simulink model "Active_mass_suspension"  (R2023a)
settings: Solver=VariableStepAuto  StartTime=0.0  StopTime=10  RelTol=1e-3
libraries: fuzblock x2, slpidlib x2, mpclib x1
settings Model: Creator=SAGNEEK SENGUPTA  LastModifiedBy=SAGNEEK SENGUPTA

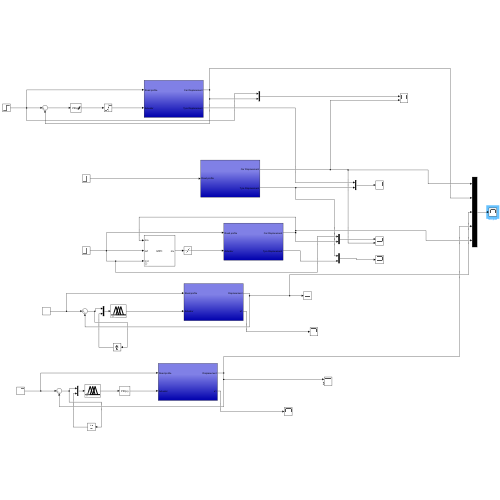
[thumbnail: Simulink's stored preview of the top-level diagram]
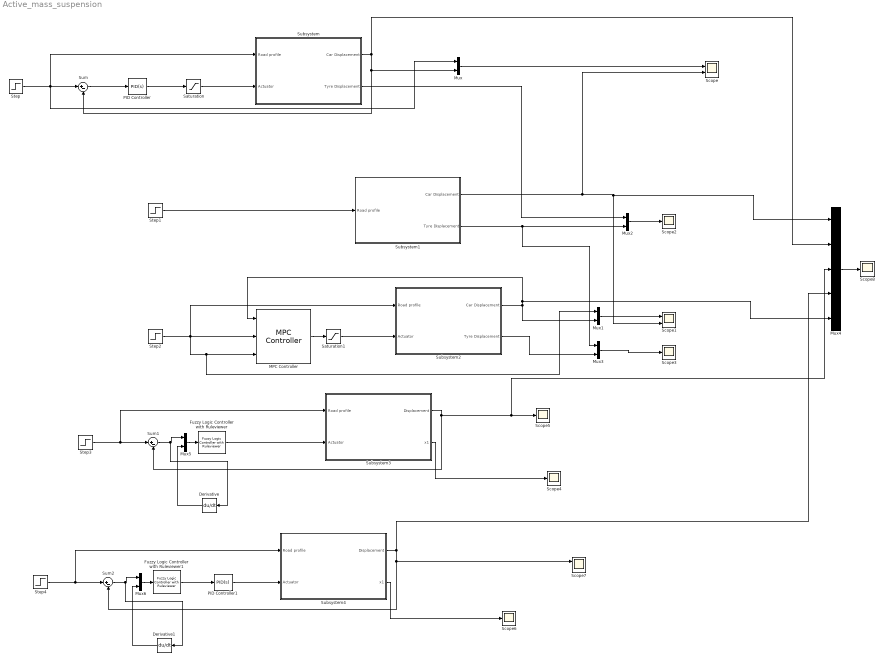
== system Active_mass_suspension ==
  Derivative : Derivative
  Derivative1 : Derivative
  Fuzzy Logic Controller with Ruleviewer : fuzblock/Fuzzy Logic  Controller  with Ruleviewer  fismatrix=rules_3  Ts=2
  Fuzzy Logic Controller with Ruleviewer1 : fuzblock/Fuzzy Logic  Controller  with Ruleviewer  fismatrix=rules_3  Ts=2
  MPC Controller : mpclib/MPC Controller  SCDEnableBlockLinearizationSpecification=on  mpcobj=mpc1  is_multiple=0  enable_value=0  return_u0=off  updateMPCinCallerWorkspace=on  md_inport=on  mv_inport=off  uref_inport=off  return_cost=off  return_mvseq=off  return_qpstatus=off  return_xseq=off  return_state=off  return_ovseq=off  state_inport=off  umin_inport=off  umax_inport=off  ymin_inport=off  ymax_inport=off  cc_inport=off  ywt_inport=off  uwt_inport=off  duwt_inport=off  rhoeps_inport=off  pm_inport=off  MaximumP=10  HorizonChoice=FixedHorizon  n_ts=0.01  n_p=12  n_mv=1  n_md=1  n_ud=0  n_mo=1  n_uo=0  BlockDataType=double  SampleTimeInherited=off  switch_inport=off
  Mux{,1..3,5..6} (6 alike) : Mux  Inputs=2
  Mux4 : Mux  Inputs=5
  PID Controller : slpidlib/PID Controller  Controller=PID  Form=Parallel  TimeDomain=Continuous-time  UseExternalTs=off  SampleTime=-1  IntegratorMethod=Forward Euler  FilterMethod=Forward Euler  ControllerParametersSource=internal  P=100  I=900  UseKiTs=on  D=80  N=1000  UseFilter=on  TunerSelectOption=Frequency Response Based  InitialConditionSource=internal  InitialConditionForIntegrator=0  InitialConditionForFilter=0  DifferentiatorICPrevScaledInput=0  ExternalReset=none  TrackingMode=off  Kt=1  LimitOutput=on  SatLimitsSource=internal  UpperSaturationLimit=800  LowerSaturationLimit=-800  LinearizeAsGain=on  AntiWindupMode=none  Kb=1  LimitIntegrator=off  UpperIntegratorSaturationLimit=inf  LowerIntegratorSaturationLimit=-inf  POutMin=[]  POutMax=[]  IOutMin=[]  IOutMax=[]  DOutMin=[]  DOutMax=[]  NOutMin=[]  NOutMax=[]  SumOutMin=[]  SumOutMax=[]  SaturationOutMin=[]  SaturationOutMax=[]  PParamMin=[]  PParamMax=[]  IParamMin=[]  IParamMax=[]  DParamMin=[]  DParamMax=[]  NParamMin=[]  NParamMax=[]  KbParamMin=[]  KbParamMax=[]  KtParamMin=[]  KtParamMax=[]  KbOutMin=[]  KbOutMax=[]  KtOutMin=[]  KtOutMax=[]  IntegratorOutMin=[]  IntegratorOutMax=[]  FilterOutMin=[]  FilterOutMax=[]  SumI1OutMin=[]  SumI1OutMax=[]  SumI2OutMin=[]  SumI2OutMax=[]  SumI3OutMin=[]  SumI3OutMax=[]  SumI4OutMin=[]  SumI4OutMax=[]  SumDOutMin=[]  SumDOutMax=[]  DifferentiatorOutMin=[]  DifferentiatorOutMax=[]  FilterDiffOutCoefMin=[]  FilterDiffOutCoefMax=[]  ReciprocalOutMin=[]  ReciprocalOutMax=[]  SumDenOutMin=[]  SumDenOutMax=[]  SumNumOutMin=[]  SumNumOutMax=[]  DivideOutMin=[]  DivideOutMax=[]  UdiffTsProdOutMin=[]  UdiffTsProdOutMax=[]  NTsProdOutMin=[]  NTsProdOutMax=[]  UintegralTsProdOutMin=[]  UintegralTsProdOutMax=[]  UngainTsProdOutMin=[]  UngainTsProdOutMax=[]  ClampingZeroOutDataTypeStr=Inherit: Inherit via back propagation  ClampingZeroOutMin=[]  ClampingZeroOutMax=[]  FilterDenConstantOutDataTypeStr=Inherit: Inherit via back propagation  FilterDenConstantOutMin=[]  FilterDenConstantOutMax=[]  PCopyOutDataTypeStr=Inherit: Inherit via back propagation  PCopyOutMin=[]  PCopyOutMax=[]  NCopyOutDataTypeStr=Inherit: Inherit via back propagation  NCopyOutMin=[]  NCopyOutMax=[]  IntegratorContinuousStateAttributes=''  IntegratorStateMustResolveToSignalObject=off  IntegratorRTWStateStorageClass=Auto  FilterContinuousStateAttributes=''  FilterStateMustResolveToSignalObject=off  FilterRTWStateStorageClass=Auto  ParallelPVariant=InternalParameters  IdealPVariant=Disabled  IVariant=InternalParameters  DVariant=InternalParameters  IntegratorVariant=Continuous  SatVariant=Enabled  AWVariant=Passthrough  PCopyVariant=Disabled  TRVariant=Disabled  FdbkBlocksVariant=Forward  IdealPFdbkVariant=Disabled  SatFdbkVariant=Disabled  DerivativeFilterVariant=ContFilter  NVariant=InternalParameters  NCopyVariant=Disabled  FilterICVariant=InternalICsFilter  IntegratorICVariant=InternalICs  ExternalResetVariant=Disabled  TRSumVariant=Passthrough  SumFdbkVariant=Disabled  SumVariant=Sum_PID  TsampFilterVariant=InternalTs  TsampNgainVariant=Passthrough  TsampIntegralVariant=Disabled_SignalSpec  ExternalSaturationOutDataTypeStr=Inherit: Same as second input
  PID Controller1 : slpidlib/PID Controller  Controller=PID  Form=Parallel  TimeDomain=Continuous-time  UseExternalTs=off  SampleTime=-1  IntegratorMethod=Forward Euler  FilterMethod=Forward Euler  ControllerParametersSource=internal  P=20  I=600  UseKiTs=off  D=0.1  N=100  UseFilter=on  TunerSelectOption=Transfer Function Based (PID Tuner App)  InitialConditionSource=internal  InitialConditionForIntegrator=0  InitialConditionForFilter=0  DifferentiatorICPrevScaledInput=0  ExternalReset=none  TrackingMode=off  Kt=1  LimitOutput=off  SatLimitsSource=internal  UpperSaturationLimit=inf  LowerSaturationLimit=-inf  LinearizeAsGain=on  AntiWindupMode=none  Kb=1  LimitIntegrator=off  UpperIntegratorSaturationLimit=inf  LowerIntegratorSaturationLimit=-inf  POutMin=[]  POutMax=[]  IOutMin=[]  IOutMax=[]  DOutMin=[]  DOutMax=[]  NOutMin=[]  NOutMax=[]  SumOutMin=[]  SumOutMax=[]  SaturationOutMin=[]  SaturationOutMax=[]  PParamMin=[]  PParamMax=[]  IParamMin=[]  IParamMax=[]  DParamMin=[]  DParamMax=[]  NParamMin=[]  NParamMax=[]  KbParamMin=[]  KbParamMax=[]  KtParamMin=[]  KtParamMax=[]  KbOutMin=[]  KbOutMax=[]  KtOutMin=[]  KtOutMax=[]  IntegratorOutMin=[]  IntegratorOutMax=[]  FilterOutMin=[]  FilterOutMax=[]  SumI1OutMin=[]  SumI1OutMax=[]  SumI2OutMin=[]  SumI2OutMax=[]  SumI3OutMin=[]  SumI3OutMax=[]  SumI4OutMin=[]  SumI4OutMax=[]  SumDOutMin=[]  SumDOutMax=[]  DifferentiatorOutMin=[]  DifferentiatorOutMax=[]  FilterDiffOutCoefMin=[]  FilterDiffOutCoefMax=[]  ReciprocalOutMin=[]  ReciprocalOutMax=[]  SumDenOutMin=[]  SumDenOutMax=[]  SumNumOutMin=[]  SumNumOutMax=[]  DivideOutMin=[]  DivideOutMax=[]  UdiffTsProdOutMin=[]  UdiffTsProdOutMax=[]  NTsProdOutMin=[]  NTsProdOutMax=[]  UintegralTsProdOutMin=[]  UintegralTsProdOutMax=[]  UngainTsProdOutMin=[]  UngainTsProdOutMax=[]  ClampingZeroOutDataTypeStr=Inherit: Inherit via back propagation  ClampingZeroOutMin=[]  ClampingZeroOutMax=[]  FilterDenConstantOutDataTypeStr=Inherit: Inherit via back propagation  FilterDenConstantOutMin=[]  FilterDenConstantOutMax=[]  PCopyOutDataTypeStr=Inherit: Inherit via back propagation  PCopyOutMin=[]  PCopyOutMax=[]  NCopyOutDataTypeStr=Inherit: Inherit via back propagation  NCopyOutMin=[]  NCopyOutMax=[]  IntegratorContinuousStateAttributes=''  IntegratorStateMustResolveToSignalObject=off  IntegratorRTWStateStorageClass=Auto  FilterContinuousStateAttributes=''  FilterStateMustResolveToSignalObject=off  FilterRTWStateStorageClass=Auto  ParallelPVariant=InternalParameters  IdealPVariant=Disabled  IVariant=InternalParameters  DVariant=InternalParameters  IntegratorVariant=Continuous  SatVariant=Disabled  AWVariant=Passthrough  PCopyVariant=Disabled  TRVariant=Disabled  FdbkBlocksVariant=Forward  IdealPFdbkVariant=Disabled  SatFdbkVariant=Disabled  DerivativeFilterVariant=ContFilter  NVariant=InternalParameters  NCopyVariant=Disabled  FilterICVariant=InternalICsFilter  IntegratorICVariant=InternalICs  ExternalResetVariant=Disabled  TRSumVariant=Passthrough  SumFdbkVariant=Disabled  SumVariant=Sum_PID  TsampFilterVariant=InternalTs  TsampNgainVariant=Passthrough  TsampIntegralVariant=Disabled_SignalSpec  ExternalSaturationOutDataTypeStr=Inherit: Same as second input
  Saturation : Saturate  UpperLimit=800  LowerLimit=-800
  Saturation1 : Saturate  UpperLimit=800  LowerLimit=-800
  Scope : Scope  NumInputPorts=2
  Scope1 : Scope  NumInputPorts=2
  Scope{2..6,8} (6 alike) : Scope
  Scope7 : Scope  NumInputPorts=2
  Step{,1..4} (5 alike) : Step  Time=0  SampleTime=0
  Subsystem : Subsystem
  Subsystem1 : Subsystem
  Subsystem2 : Subsystem
  Subsystem3 : Subsystem
  Subsystem4 : Subsystem
  Sum : Sum  Inputs=|+-
  Sum1 : Sum  Inputs=|+-
  Sum2 : Sum  Inputs=|+-
  wires:
  Step/1 -> Subsystem/1(Road profile), Sum/1, Mux/1
  Saturation/1 -> Subsystem/2(Actuator)
  Subsystem/1(Car Displacement) -> Sum/2, Mux/2, Mux4/2
  Mux/1 -> Scope/1
  Step1/1 -> Subsystem1/1(Road profile)
  Subsystem1/1(Car Displacement) -> Mux4/1, Scope1/2, Scope/2
  PID Controller/1 -> Saturation/1
  Sum/1 -> PID Controller/1
  Saturation1/1 -> Subsystem2/2(Actuator)
  Subsystem2/1(Car Displacement) -> Mux1/2, Mux4/5, MPC Controller/1
  Mux1/1 -> Scope1/1
  MPC Controller/1 -> Saturation1/1
  Step2/1 -> MPC Controller/2, Mux1/1, MPC Controller/3, Subsystem2/1(Road profile)
  Subsystem1/2(Tyre Displacement) -> Mux3/1, Mux2/2
  Subsystem/2(Tyre Displacement) -> Mux2/1
  Mux2/1 -> Scope2/1
  Subsystem2/2(Tyre Displacement) -> Mux3/2
  Mux3/1 -> Scope3/1
  Subsystem4/1(Displacement) -> Scope7/1, Sum2/2, Mux4/4
  Derivative1/1 -> Mux6/2
  Step4/1 -> Subsystem4/1(Road profile), Sum2/1
  Mux6/1 -> Fuzzy Logic Controller with Ruleviewer1/1
  Fuzzy Logic Controller with Ruleviewer1/1 -> PID Controller1/1
  PID Controller1/1 -> Subsystem4/2(Actuator)
  Sum2/1 -> Derivative1/1, Mux6/1
  Subsystem4/2(x1) -> Scope6/1
  Fuzzy Logic Controller with Ruleviewer/1 -> Subsystem3/2(Actuator)
  Subsystem3/2(x1) -> Scope4/1
  Step3/1 -> Subsystem3/1(Road profile), Sum1/1
  Subsystem3/1(Displacement) -> Mux4/3, Scope5/1, Sum1/2
  Derivative/1 -> Mux5/2
  Sum1/1 -> Derivative/1, Mux5/1
  Mux5/1 -> Fuzzy Logic Controller with Ruleviewer/1
  Mux4/1 -> Scope8/1

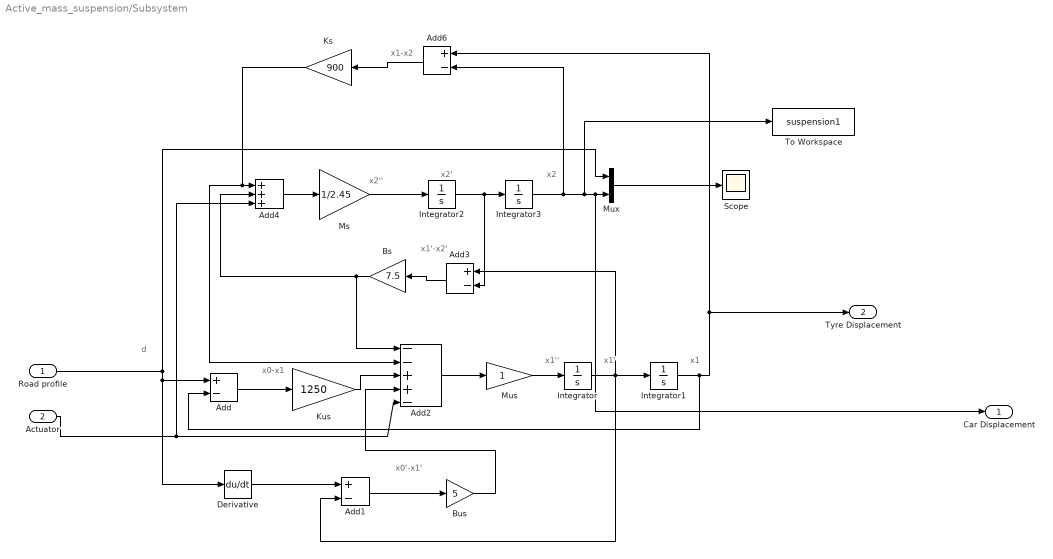
== system Active_mass_suspension/Subsystem ==
  note: x0-x1
  note: x0'-x1'
  note: x1
  note: x1'
  note: x2'
  note: x2''
  note: d
  note: x1'-x2'
  note: x1-x2
  note: x2
  note: x1''
  Road profile : Inport
  Actuator : Inport  Port=2
  Add{,1,3,6} (4 alike) : Sum  Inputs=+-
  Add2 : Sum  Inputs=--++-
  Add4 : Sum  Inputs=+++
  Bs : Gain  Gain=7.5
  Bus : Gain  Gain=5
  Derivative : Derivative
  Integrator{,1..3} (4 alike) : Integrator
  Ks : Gain  Gain=900
  Kus : Gain  Gain=1250
  Ms : Gain  Gain=1/2.45
  Mus : Gain
  Mux : Mux  Inputs=2
  Scope : Scope
  To Workspace : ToWorkspace  VariableName=suspension1  SaveFormat=Timeseries  SampleTime=-1
  Car Displacement : Outport
  Tyre Displacement : Outport  Port=2
  wires:
  Integrator1/1 -> Add/2, Tyre Displacement/1, Add6/1
  Bs/1 -> Add4/2, Add2/1
  Ms/1 -> Integrator2/1
  Bus/1 -> Add2/4
  Actuator/1 -> Add4/3, Add2/5
  Kus/1 -> Add2/3
  Integrator3/1 -> Car Displacement/1, Mux/2, To Workspace/1, Add6/2
  Add/1 -> Kus/1
  Mus/1 -> Integrator/1
  Ks/1 -> Add2/2, Add4/1
  Mux/1 -> Scope/1
  Add3/1 -> Bs/1
  Integrator2/1 -> Add3/2, Integrator3/1
  Add1/1 -> Bus/1
  Derivative/1 -> Add1/1
  Add2/1 -> Mus/1
  Integrator/1 -> Add1/2, Add3/1, Integrator1/1
  Add4/1 -> Ms/1
  Road profile/1 -> Derivative/1, Add/1, Mux/1
  Add6/1 -> Ks/1

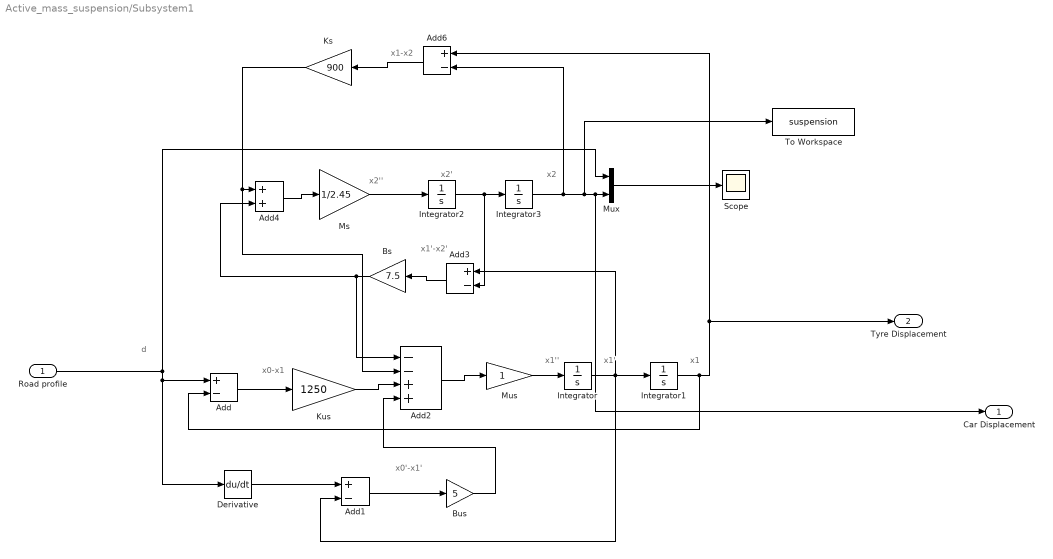
== system Active_mass_suspension/Subsystem1 ==
  note: x0-x1
  note: x0'-x1'
  note: x1
  note: x1'
  note: x2'
  note: x2''
  note: d
  note: x1'-x2'
  note: x1-x2
  note: x2
  note: x1''
  Road profile : Inport
  Add{,1,3,6} (4 alike) : Sum  Inputs=+-
  Add2 : Sum  Inputs=--++
  Add4 : Sum
  Bs : Gain  Gain=7.5
  Bus : Gain  Gain=5
  Derivative : Derivative
  Integrator{,1..3} (4 alike) : Integrator
  Ks : Gain  Gain=900
  Kus : Gain  Gain=1250
  Ms : Gain  Gain=1/2.45
  Mus : Gain
  Mux : Mux  Inputs=2
  Scope : Scope
  To Workspace : ToWorkspace  VariableName=suspension  SaveFormat=Timeseries  SampleTime=-1
  Car Displacement : Outport
  Tyre Displacement : Outport  Port=2
  wires:
  Integrator1/1 -> Add/2, Tyre Displacement/1, Add6/1
  Bs/1 -> Add4/2, Add2/1
  Ms/1 -> Integrator2/1
  Bus/1 -> Add2/4
  Kus/1 -> Add2/3
  Integrator3/1 -> Car Displacement/1, Mux/2, To Workspace/1, Add6/2
  Add/1 -> Kus/1
  Mus/1 -> Integrator/1
  Ks/1 -> Add2/2, Add4/1
  Mux/1 -> Scope/1
  Add3/1 -> Bs/1
  Integrator2/1 -> Add3/2, Integrator3/1
  Add1/1 -> Bus/1
  Derivative/1 -> Add1/1
  Add2/1 -> Mus/1
  Integrator/1 -> Add1/2, Add3/1, Integrator1/1
  Add4/1 -> Ms/1
  Road profile/1 -> Derivative/1, Add/1, Mux/1
  Add6/1 -> Ks/1

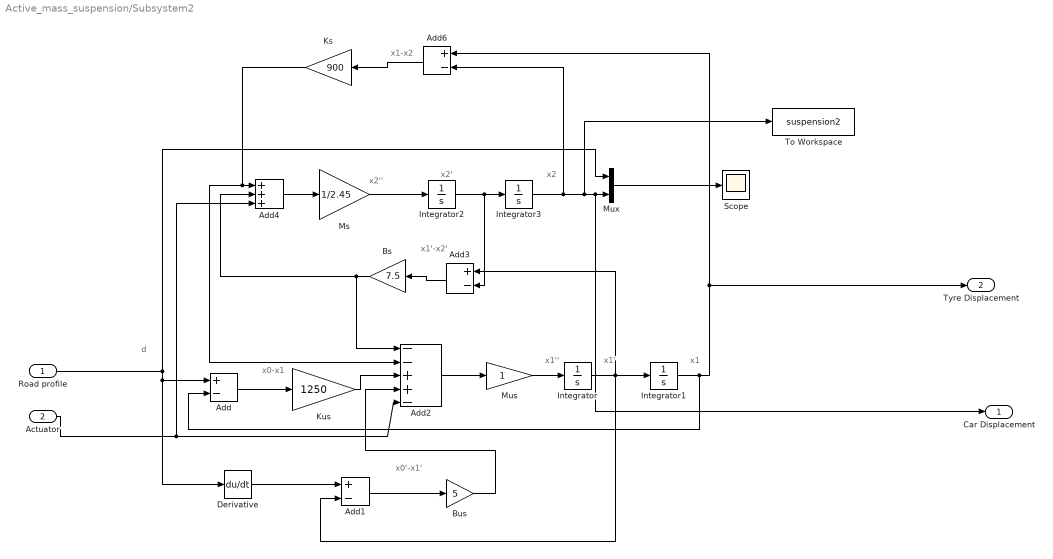
== system Active_mass_suspension/Subsystem2 ==
  note: x0-x1
  note: x0'-x1'
  note: x1
  note: x1'
  note: x2'
  note: x2''
  note: d
  note: x1'-x2'
  note: x1-x2
  note: x2
  note: x1''
  Road profile : Inport
  Actuator : Inport  Port=2
  Add{,1,3,6} (4 alike) : Sum  Inputs=+-
  Add2 : Sum  Inputs=--++-
  Add4 : Sum  Inputs=+++
  Bs : Gain  Gain=7.5
  Bus : Gain  Gain=5
  Derivative : Derivative
  Integrator{,1..3} (4 alike) : Integrator
  Ks : Gain  Gain=900
  Kus : Gain  Gain=1250
  Ms : Gain  Gain=1/2.45
  Mus : Gain
  Mux : Mux  Inputs=2
  Scope : Scope
  To Workspace : ToWorkspace  VariableName=suspension2  SaveFormat=Timeseries  SampleTime=-1
  Car Displacement : Outport
  Tyre Displacement : Outport  Port=2
  wires:
  Integrator1/1 -> Add/2, Tyre Displacement/1, Add6/1
  Bs/1 -> Add4/2, Add2/1
  Ms/1 -> Integrator2/1
  Bus/1 -> Add2/4
  Actuator/1 -> Add4/3, Add2/5
  Kus/1 -> Add2/3
  Integrator3/1 -> Car Displacement/1, Mux/2, To Workspace/1, Add6/2
  Add/1 -> Kus/1
  Mus/1 -> Integrator/1
  Ks/1 -> Add2/2, Add4/1
  Mux/1 -> Scope/1
  Add3/1 -> Bs/1
  Integrator2/1 -> Add3/2, Integrator3/1
  Add1/1 -> Bus/1
  Derivative/1 -> Add1/1
  Add2/1 -> Mus/1
  Integrator/1 -> Add1/2, Add3/1, Integrator1/1
  Add4/1 -> Ms/1
  Road profile/1 -> Derivative/1, Add/1, Mux/1
  Add6/1 -> Ks/1

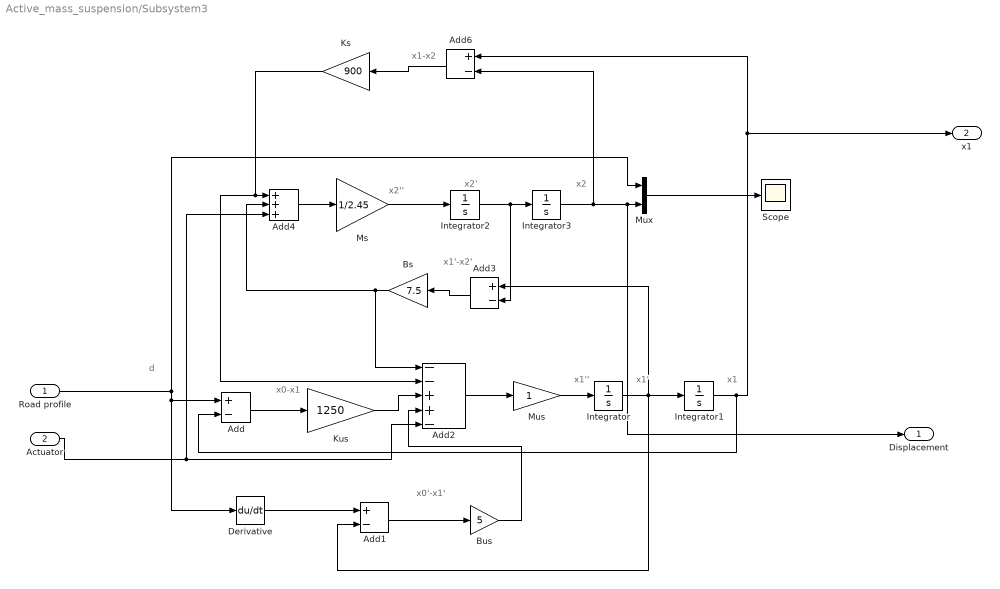
== system Active_mass_suspension/Subsystem3 ==
  note: x0-x1
  note: x0'-x1'
  note: x1
  note: x1'
  note: x2'
  note: x2''
  note: d
  note: x1'-x2'
  note: x1-x2
  note: x2
  note: x1''
  Road profile : Inport
  Actuator : Inport  Port=2
  Add{,1,3,6} (4 alike) : Sum  Inputs=+-
  Add2 : Sum  Inputs=--++-
  Add4 : Sum  Inputs=+++
  Bs : Gain  Gain=7.5
  Bus : Gain  Gain=5
  Derivative : Derivative
  Integrator{,1..3} (4 alike) : Integrator
  Ks : Gain  Gain=900
  Kus : Gain  Gain=1250
  Ms : Gain  Gain=1/2.45
  Mus : Gain
  Mux : Mux  Inputs=2
  Scope : Scope
  Displacement : Outport
  x1 : Outport  Port=2
  wires:
  Integrator1/1 -> Add/2, x1/1, Add6/1
  Bs/1 -> Add4/2, Add2/1
  Ms/1 -> Integrator2/1
  Bus/1 -> Add2/4
  Actuator/1 -> Add4/3, Add2/5
  Kus/1 -> Add2/3
  Integrator3/1 -> Displacement/1, Mux/2, Add6/2
  Add/1 -> Kus/1
  Mus/1 -> Integrator/1
  Ks/1 -> Add2/2, Add4/1
  Mux/1 -> Scope/1
  Add3/1 -> Bs/1
  Integrator2/1 -> Add3/2, Integrator3/1
  Add1/1 -> Bus/1
  Derivative/1 -> Add1/1
  Add2/1 -> Mus/1
  Integrator/1 -> Add1/2, Add3/1, Integrator1/1
  Add4/1 -> Ms/1
  Road profile/1 -> Derivative/1, Add/1, Mux/1
  Add6/1 -> Ks/1

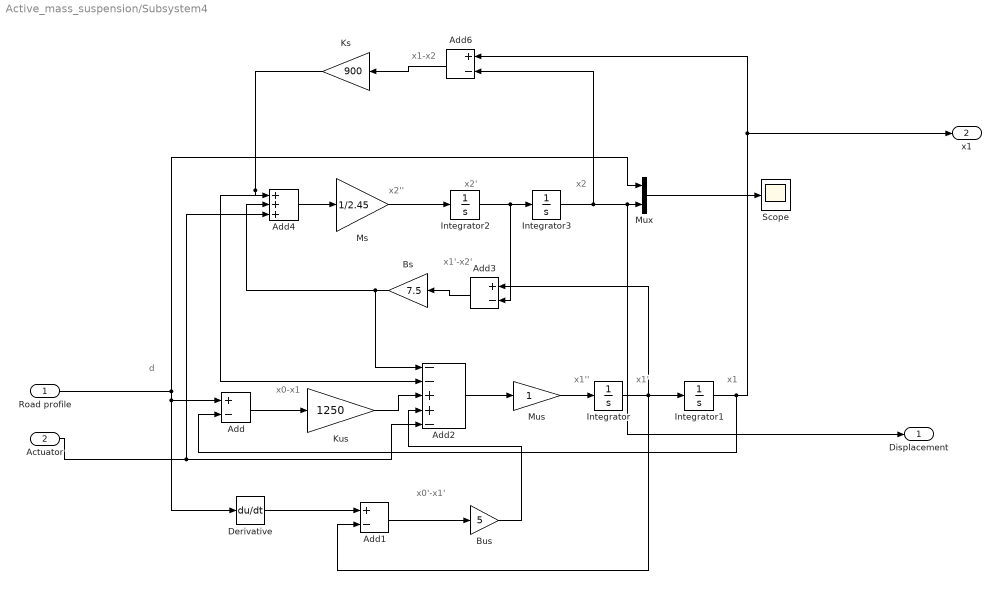
== system Active_mass_suspension/Subsystem4 ==
  note: x0-x1
  note: x0'-x1'
  note: x1
  note: x1'
  note: x2'
  note: x2''
  note: d
  note: x1'-x2'
  note: x1-x2
  note: x2
  note: x1''
  Road profile : Inport
  Actuator : Inport  Port=2
  Add{,1,3,6} (4 alike) : Sum  Inputs=+-
  Add2 : Sum  Inputs=--++-
  Add4 : Sum  Inputs=+++
  Bs : Gain  Gain=7.5
  Bus : Gain  Gain=5
  Derivative : Derivative
  Integrator{,1..3} (4 alike) : Integrator
  Ks : Gain  Gain=900
  Kus : Gain  Gain=1250
  Ms : Gain  Gain=1/2.45
  Mus : Gain
  Mux : Mux  Inputs=2
  Scope : Scope
  Displacement : Outport
  x1 : Outport  Port=2
  wires:
  Integrator1/1 -> Add/2, x1/1, Add6/1
  Bs/1 -> Add4/2, Add2/1
  Ms/1 -> Integrator2/1
  Bus/1 -> Add2/4
  Actuator/1 -> Add4/3, Add2/5
  Kus/1 -> Add2/3
  Integrator3/1 -> Displacement/1, Mux/2, Add6/2
  Add/1 -> Kus/1
  Mus/1 -> Integrator/1
  Ks/1 -> Add2/2, Add4/1
  Mux/1 -> Scope/1
  Add3/1 -> Bs/1
  Integrator2/1 -> Add3/2, Integrator3/1
  Add1/1 -> Bus/1
  Derivative/1 -> Add1/1
  Add2/1 -> Mus/1
  Integrator/1 -> Add1/2, Add3/1, Integrator1/1
  Add4/1 -> Ms/1
  Road profile/1 -> Derivative/1, Add/1, Mux/1
  Add6/1 -> Ks/1
